simulink model "noisyTheta"  (Simulink 7.6)
settings: Solver=ode45  StartTime=0.0  StopTime=200  RelTol=1e-3
libraries: simulink x4, fuzblock x1, commnoisgen2 x1
settings Model: Creator=ASUS  LastModifiedBy=ASUS

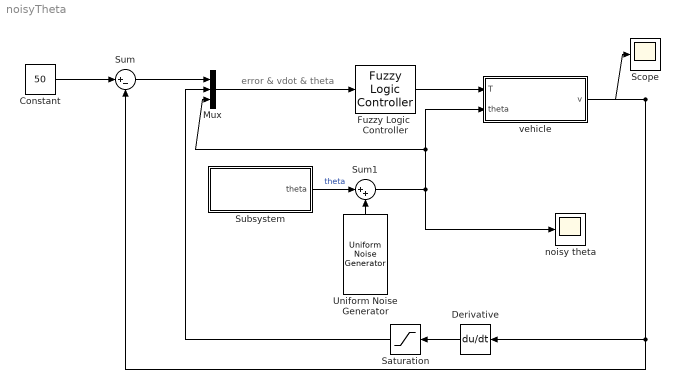
== system noisyTheta ==
  note: error & vdot & theta
  Constant : Constant  Value=50
  Derivative : Derivative
  Fuzzy Logic  Controller : fuzblock/Fuzzy Logic  Controller  SystemSampleTime=-1  fis='vehicle'
  Mux : Mux  Inputs=3
  Saturation : Saturate
  Scope : Scope
      settings: YMin=0  YMax=50
  Subsystem : Subsystem
  Sum : Sum  Inputs=|+-
  Sum1 : Sum  Inputs=|++
  Uniform Noise Generator : commnoisgen2/Uniform Noise Generator  SystemSampleTime=-1  low=-2  up=2  seed=31  Ts=1  frameBased=off  sampPerFrame=1  orient=off  outDataType=double
  noisy theta : Scope
      settings: YMin=0  YMax=50  SaveName=ScopeData2
  vehicle : Subsystem
  wires:
  vehicle/1(v) -> Derivative/1, Sum/2, Scope/1
  Derivative/1 -> Saturation/1
  Mux/1 -> Fuzzy Logic  Controller/1
  Saturation/1 -> Mux/2
  Sum/1 -> Mux/1
  Constant/1 -> Sum/1
  Fuzzy Logic  Controller/1 -> vehicle/1(T)
  Subsystem/1(theta) -> Sum1/1  "theta"
  Uniform Noise Generator/1 -> Sum1/2
  Sum1/1 -> noisy theta/1, vehicle/2(theta), Mux/3

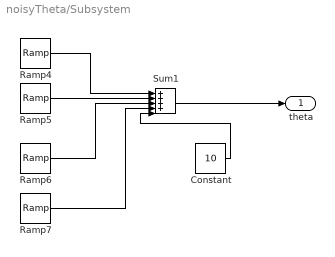
== system noisyTheta/Subsystem ==
  Constant : Constant  Value=10
  Ramp4 : simulink/Sources/Ramp  SystemSampleTime=-1  slope=.25  start=0  X0=-5
  Ramp5 : simulink/Sources/Ramp  SystemSampleTime=-1  slope=-.25  start=20  X0=0
  Ramp6 : simulink/Sources/Ramp  SystemSampleTime=-1  slope=0.25  start=40  X0=0
  Ramp7 : simulink/Sources/Ramp  SystemSampleTime=-1  slope=-.25  start=80  X0=10
  Sum1 : Sum  Inputs=|++++-
  theta : Outport
  wires:
  Ramp4/1 -> Sum1/1
  Ramp5/1 -> Sum1/2
  Ramp6/1 -> Sum1/3
  Ramp7/1 -> Sum1/4
  Constant/1 -> Sum1/5
  Sum1/1 -> theta/1

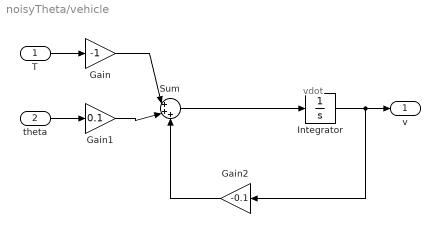
== system noisyTheta/vehicle ==
  note: vdot
  T : Inport
  theta : Inport  Port=2
  Gain : Gain  Gain=-1
  Gain1 : Gain  Gain=0.1
  Gain2 : Gain  Gain=-0.1
  Integrator : Integrator
  Sum : Sum  Inputs=|+++
  v : Outport
  wires:
  T/1 -> Gain/1
  theta/1 -> Gain1/1
  Gain/1 -> Sum/1
  Gain1/1 -> Sum/2
  Integrator/1 -> v/1, Gain2/1
  Sum/1 -> Integrator/1
  Gain2/1 -> Sum/3
